simulink model "Avoid_vat_can_3xe"  (R2021b)
settings: Solver=FixedStepAuto  StartTime=0.0  StopTime=40  FixedStep=0.01  RelTol=1e-3
values from neighbouring files (symbols this model uses):
  G_target = [5.8;8.0]    [parameter.m]
  Position_first_vehicle = [Set_first(1);Set_first(2);deg2rad(19.5)]    [parameter.m]
  Q_can = [4.4;7.2]    [parameter.m]
  Set_first = [3;6]    [parameter.m]
settings Model: Creator=HL_1810  LastModifiedBy=HL_1810

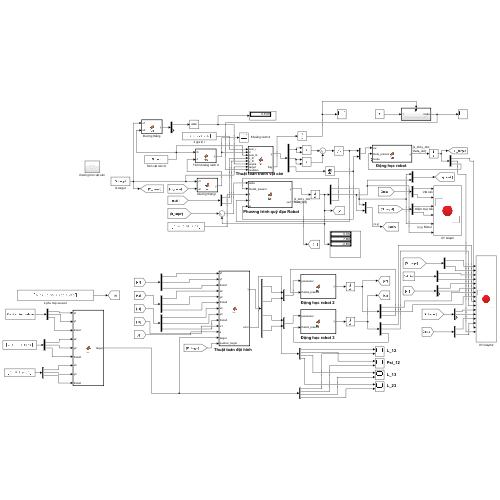
[thumbnail: Simulink's stored preview of the top-level diagram]
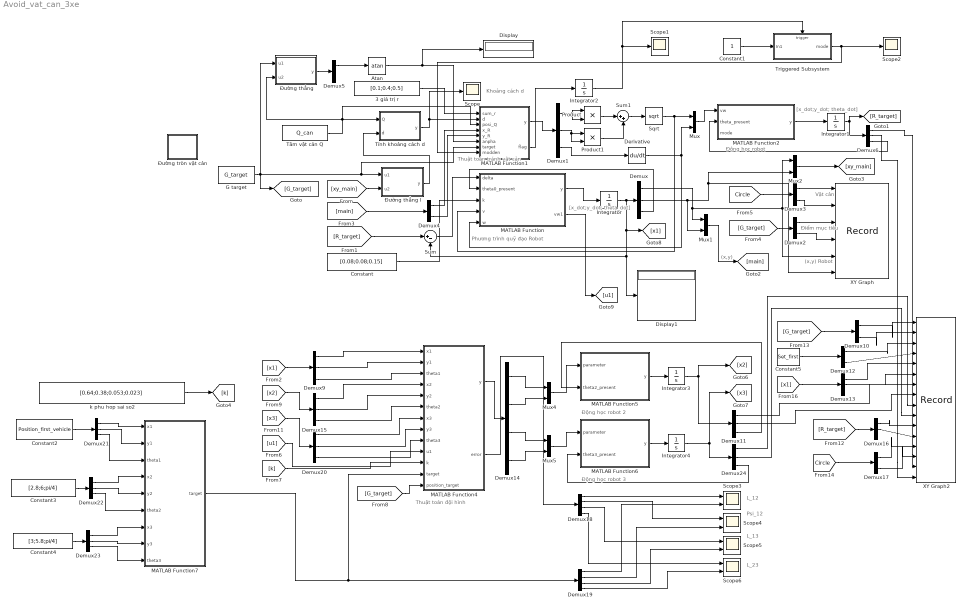
== system Avoid_vat_can_3xe ==
  note: (x,y)
  note: Điểm mục tiêu
  note: (x,y) Robot
  note: Động học robot
  note: Khoảng cách d
  note: Phương trình quỹ đạo Robot
  note: Thuật toán tránh vật cản
  note: Vật cản
  note: [x_dot;y_dot;
      | theta_dot]
  note: [x_dot;y_dot;
      | theta_dot]
  note: L_12
  note: Psi_12
  note: Động học robot 3
  note: L_13
  note: Động học robot 2
  note: L_23
  note: Thuật toán đội hình
  3 giá trị r : Constant  Value=[0.1;0.4;0.5]
  Atan : Trigonometry  Operator=atan
  Constant : Constant  Value=[0.08;0.08;0.15]
  Constant1 : Constant
  Constant2 : Constant  Value=Position_first_vehicle
  Constant3 : Constant  Value=[2.8;6;pi/4]
  Constant4 : Constant  Value=[3;5.8;pi/4]
  Constant5 : Constant  Value=Set_first
  Demux{,1,6,9,11,13,15..16,20..24} (13 alike) : Demux  Outputs=3
  Demux{2..5,10,12,17} (7 alike) : Demux  Outputs=2
  Demux14 : Demux
  Demux18 : Demux
  Demux19 : Demux
  Derivative : Derivative
  Display : Display
  Display1 : Display
  G target : Constant  Value=G_target
  Integrator : Integrator  InitialCondition=Position_first_vehicle
  Integrator1 : Integrator  InitialCondition=Position_first_vehicle
  Integrator2 : Integrator
  Integrator3 : Integrator  InitialCondition=[2.8;6;pi/4]
  Integrator4 : Integrator  InitialCondition=[3;5.8;pi/4]
  MATLAB Function : MATLAB Function  TreatAsAtomicUnit=on
  MATLAB Function1 : MATLAB Function  TreatAsAtomicUnit=on
  MATLAB Function2 : MATLAB Function  TreatAsAtomicUnit=on
  MATLAB Function4 : MATLAB Function  TreatAsAtomicUnit=on
  MATLAB Function5 : MATLAB Function  TreatAsAtomicUnit=on
  MATLAB Function6 : MATLAB Function  TreatAsAtomicUnit=on
  MATLAB Function7 : MATLAB Function  TreatAsAtomicUnit=on
  Mux{,1..2,4..5} (5 alike) : Mux  Inputs=2
  Product : Product
  Product1 : Product
  Scope : Scope
  Scope1 : Scope
  Scope2 : Scope
  Scope{3..6} (4 alike) : Scope  NumInputPorts=2
  Sqrt : Sqrt  SaturateOnIntegerOverflow=on
  Sum : Sum  Inputs=|+-
  Sum1 : Sum  Inputs=|++
  Triggered Subsystem : Subsystem  TreatAsAtomicUnit=on
  Tâm vật cản Q : Constant  Value=Q_can
  Tính khoảng cách d : MATLAB Function  TreatAsAtomicUnit=on
  XY Graph : Record  FileSettingsInternal="{\"entries\":[{\"content\":{\"excelSettings\":{\"content\":{},\"type\":\"Streamout.ExcelSettings\"}},\"type\":\"Streamout.FileSettingStorage\",\"uuid\":\"a8d3b570-9e37-41a1-b9b1-4b418e9d51ca\"}],\"packageUris\":[\"http://schema.mathworks.com/mf0/streamout_blocks/R2020a\"],\"version\":\"1.0\"}"  Layout=[1 1]  SignalsInternal="{\"entries\":[{\"content\":{\"signals\":[{\"content\":{\"blockPath\":[\"Avoid_vat_can_3xe/XY Graph\"],\"channel\":[],\"dimensions\":[1],\"domain\":\"Avoid_vat_can_3xe/XY Graph\",\"lineColor\":\"#ff6929\",\"plots\":[1],\"port\":1,\"sid\":[\"\"],\"signalID\":4338,\"signalName\":\"Demux3:1\"},\"type\":\"RecordBlkView.Signal\",\"uuid\":\"8399b9d0-b1dd-4b64-90be-267014180888\"},{\"content\":{\"blockPath\":[\"Avoid_vat_can_3xe/XY Graph\"],\"channel\":[],\"dimensions\":[1],\"domain\":\"Avoid_vat_can_3xe/XY Graph\",\"lineColor\":\"#b746ff\",\"plots\":[1],\"port\":2,\"sid\":[\"\"],\"signalID\":4342,\"signalName\":\"Demux3:2\"},\"type\":\"RecordBlkView.Signal\",\"uuid\":\"5d023b2a-6e03-4b3e-9db3-6ad99874a4d7\"},{\"content\":{\"blockPath\":[\"Avoid_vat_can_3xe/XY Graph\"],\"channel\":[],\"dimensions\":[1],\"domain\":\"Avoid_vat_can_3xe/XY Graph\",\"lineColor\":\"#64d413\",\"plots\":[1],\"port\":5,\"sid\":[\"\"],\"signalID\":4346,\"signalName\":\"Demux:1\"},\"type\":\"RecordBlkView.Signal\",\"uuid\":\"95680c87-e324-4348-a78d-b81f180a8f94\"},{\"content\":{\"blockPath\":[\"Avoid_vat_can_3xe/XY Graph\"],\"channel\":[],\"dimensions\":[1],\"domain\":\"Avoid_vat_can_3xe/XY Graph\",\"lineColor\":\"#ff13a6\",\"plots\":[1],\"port\":6,\"sid\":[\"\"],\"signalID\":4350,\"signalName\":\"Demux:2\"},\"type\":\"RecordBlkView.Signal\",\"uuid\":\"adc273e3-6312-475d-85d5-afca6bf7d5e4\"},{\"content\":{\"blockPath\":[\"Avoid_vat_can_3xe/XY Graph\"],\"channel\":[],\"dimensions\":[1],\"domain\":\"Avoid_vat_can_3xe/XY Graph\",\"lineColor\":\"#fe330a\",\"plots\":[1],\"port\":3,\"sid\":[\"\"],\"signalID\":4402,\"signalName\":\"Demux2:1\"},\"type\":\"RecordBlkView.Signal\",\"uuid\":\"c6965b63-4477-498a-81ce-133a2781b2ed\"},{\"content\":{\"blockPath\":[\"Avoid_vat_can_3xe/XY Graph\"],\"channel\":[],\"dimensions\":[1],\"domain\":\"Avoid_vat_can_3xe/XY Graph\",\"lineColor\":\"#22b573\",\"plots\":[1],\"port\":4,\"sid\":[\"\"],\"signalID\":4406,\"signalName\":\"Demux2:2\"},\"type\":\"RecordBlkView.Signal\",\"uuid\":\"82515902-e219-45b4-8869-39249660641d\"}]},\"type\":\"RecordBlkView.InputSignals\",\"uuid\":\"3ec44429-ff9f-4d5f-a42a-4439dbfec8c0\"}],\"packageUris\":[\"http://schema.mathworks.com/mf0/streamout_blocks/R2020a\"],\"version\":\"1.0\"}"  VisualizationBindings="{\"xyplotplugin\":{\"info\":[{\"series\":[{\"bindingParametersList\":[{\"parameter\":\"X-Axis\",\"signalID\":4338,\"signalName\":\"Demux3:1\"},{\"parameter\":\"Y-Axis\",\"signalID\":4342,\"signalName\":\"Demux3:2\"}],\"seriesID\":26607},{\"bindingParametersList\":[{\"parameter\":\"X-Axis\",\"signalID\":4402,\"signalName\":\"Demux2:1\"},{\"parameter\":\"Y-Axis\",\"signalID\":4406,\"signalName\":\"Demux2:2\"}],\"seriesID\":58074},{\"bindingParametersList\":[{\"parameter\":\"X-Axis\",\"signalID\":4346,\"signalName\":\"Demux:1\"},{\"parameter\":\"Y-Axis\",\"signalID\":4350,\"signalName\":\"Demux:2\"}],\"seriesID\":51744}],\"subplotID\":1},{\"series\":[],\"subplotID\":2}]}}"  CompatibilityTag=XY
  XY Graph2 : Record  FileSettingsInternal="{\"entries\":[{\"content\":{\"excelSettings\":{\"content\":{},\"type\":\"Streamout.ExcelSettings\"}},\"type\":\"Streamout.FileSettingStorage\",\"uuid\":\"ed37455e-9adf-4e9b-bed2-b0034767e237\"}],\"packageUris\":[\"http://schema.mathworks.com/mf0/streamout_blocks/R2020a\"],\"version\":\"1.0\"}"  Layout=[1 1]  SignalsInternal="{\"entries\":[{\"content\":{\"signals\":[{\"content\":{\"blockPath\":[\"Avoid_vat_can_3xe/XY Graph2\"],\"channel\":[],\"dimensions\":[1],\"domain\":\"Avoid_vat_can_3xe/XY Graph2\",\"lineColor\":\"#ff6929\",\"plots\":[1],\"port\":5,\"sid\":[\"\"],\"signalID\":4354,\"signalName\":\"Demux13:1\"},\"type\":\"RecordBlkView.Signal\",\"uuid\":\"0d8b8474-356b-455b-a3d2-928f594b97db\"},{\"content\":{\"blockPath\":[\"Avoid_vat_can_3xe/XY Graph2\"],\"channel\":[],\"dimensions\":[1],\"domain\":\"Avoid_vat_can_3xe/XY Graph2\",\"lineColor\":\"#b746ff\",\"plots\":[1],\"port\":6,\"sid\":[\"\"],\"signalID\":4358,\"signalName\":\"Demux13:2\"},\"type\":\"RecordBlkView.Signal\",\"uuid\":\"c7b2e1ea-afc6-4af0-a64e-b0961d81559b\"},{\"content\":{\"blockPath\":[\"Avoid_vat_can_3xe/XY Graph2\"],\"channel\":[],\"dimensions\":[1,1],\"domain\":\"Avoid_vat_can_3xe/XY Graph2\",\"lineColor\":\"#64d413\",\"plots\":[1],\"port\":7,\"sid\":[\"\"],\"signalID\":4362,\"signalName\":\"Demux11:1\"},\"type\":\"RecordBlkView.Signal\",\"uuid\":\"9d6d36d3-8fd9-4190-aa51-39a149636880\"},{\"content\":{\"blockPath\":[\"Avoid_vat_can_3xe/XY Graph2\"],\"channel\":[],\"dimensions\":[1,1],\"domain\":\"Avoid_vat_can_3xe/XY Graph2\",\"lineColor\":\"#ff13a6\",\"plots\":[1],\"port\":8,\"sid\":[\"\"],\"signalID\":4366,\"signalName\":\"Demux11:2\"},\"type\":\"RecordBlkView.Signal\",\"uuid\":\"809edec6-6648-46b3-b799-dc7e2610b91b\"},{\"content\":{\"blockPath\":[\"Avoid_vat_can_3xe/XY Graph2\"],\"channel\":[],\"dimensions\":[1,1],\"domain\":\"Avoid_vat_can_3xe/XY Graph2\",\"lineColor\":\"#fe330a\",\"plots\":[1],\"port\":9,\"sid\":[\"\"],\"signalID\":4370,\"signalName\":\"Demux24:1\"},\"type\":\"RecordBlkView.Signal\",\"uuid\":\"bc8e87cb-6b4d-42b2-8550-ea17e29acf2f\"},{\"content\":{\"blockPath\":[\"Avoid_vat_can_3xe/XY Graph2\"],\"channel\":[],\"dimensions\":[1,1],\"domain\":\"Avoid_vat_can_3xe/XY Graph2\",\"lineColor\":\"#22b573\",\"plots\":[1],\"port\":10,\"sid\":[\"\"],\"signalID\":4374,\"signalName\":\"Demux24:2\"},\"type\":\"RecordBlkView.Signal\",\"uuid\":\"436826c5-510a-4675-9b17-c630ed9073da\"},{\"content\":{\"blockPath\":[\"Avoid_vat_can_3xe/XY Graph2\"],\"channel\":[],\"dimensions\":[1],\"domain\":\"Avoid_vat_can_3xe/XY Graph2\",\"lineColor\":\"#0072bd\",\"plots\":[1],\"port\":11,\"sid\":[\"\"],\"signalID\":4378,\"signalName\":\"Demux16:1\"},\"type\":\"RecordBlkView.Signal\",\"uuid\":\"45a9fc4d-343a-4103-b6bd-5c0be15f774b\"},{\"content\":{\"blockPath\":[\"Avoid_vat_can_3xe/XY Graph2\"],\"channel\":[],\"dimensions\":[1],\"domain\":\"Avoid_vat_can_3xe/XY Graph2\",\"lineColor\":\"#d95319\",\"plots\":[1],\"port\":12,\"sid\":[\"\"],\"signalID\":4382,\"signalName\":\"Demux16:2\"},\"type\":\"RecordBlkView.Signal\",\"uuid\":\"679dac8d-d637-4fab-bff7-509533d3bec0\"},{\"content\":{\"blockPath\":[\"Avoid_vat_can_3xe/XY Graph2\"],\"channel\":[],\"dimensions\":[1],\"domain\":\"Avoid_vat_can_3xe/XY Graph2\",\"lineColor\":\"#fe330a\",\"plots\":[1],\"port\":13,\"sid\":[\"\"],\"signalID\":4386,\"signalName\":\"Demux17:1\"},\"type\":\"RecordBlkView.Signal\",\"uuid\":\"4ab9b0f9-b6f9-4618-a1ff-eb8b4a502663\"},{\"content\":{\"blockPath\":[\"Avoid_vat_can_3xe/XY Graph2\"],\"channel\":[],\"dimensions\":[1],\"domain\":\"Avoid_vat_can_3xe/XY Graph2\",\"lineColor\":\"#22b573\",\"plots\":[1],\"port\":14,\"sid\":[\"\"],\"signalID\":4390,\"signalName\":\"Demux17:2\"},\"type\":\"RecordBlkView.Signal\",\"uuid\":\"5823eff9-447f-4ca4-82e1-f72dafea7aa2\"},{\"content\":{\"blockPath\":[\"Avoid_vat_can_3xe/XY Graph2\"],\"channel\":[],\"dimensions\":[1],\"domain\":\"Avoid_vat_can_3xe/XY Graph2\",\"lineColor\":\"#64d413\",\"plots\":[1],\"port\":15,\"sid\":[\"\"],\"signalID\":4394,\"signalName\":\"Demux6:1\"},\"type\":\"RecordBlkView.Signal\",\"uuid\":\"6e0b1d86-1497-48ad-b697-da4d1b4b05da\"},{\"content\":{\"blockPath\":[\"Avoid_vat_can_3xe/XY Graph2\"],\"channel\":[],\"dimensions\":[1],\"domain\":\"Avoid_vat_can_3xe/XY Graph2\",\"lineColor\":\"#ff13a6\",\"plots\":[1],\"port\":16,\"sid\":[\"\"],\"signalID\":4398,\"signalName\":\"Demux6:2\"},\"type\":\"RecordBlkView.Signal\",\"uuid\":\"a773829a-94af-4e1e-bb77-84491575b248\"},{\"content\":{\"blockPath\":[\"Avoid_vat_can_3xe/XY Graph2\"],\"channel\":[],\"dimensions\":[1],\"domain\":\"Avoid_vat_can_3xe/XY Graph2\",\"lineColor\":\"#77ac30\",\"plots\":[1],\"port\":1,\"sid\":[\"\"],\"signalID\":4410,\"signalName\":\"Demux10:1\"},\"type\":\"RecordBlkView.Signal\",\"uuid\":\"59508f2c-7fd3-4530-ba17-a0911d246959\"},{\"content\":{\"blockPath\":[\"Avoid_vat_can_3xe/XY Graph2\"],\"channel\":[],\"dimensions\":[1],\"domain\":\"Avoid_vat_can_3xe/XY Graph2\",\"lineColor\":\"#4dbeee\",\"plots\":[1],\"port\":2,\"sid\":[\"\"],\"signalID\":4414,\"signalName\":\"Demux10:2\"},\"type\":\"RecordBlkView.Signal\",\"uuid\":\"ec991bf2-35d2-4910-97d5-0e3210c8fdc5\"},{\"content\":{\"blockPath\":[\"Avoid_vat_can_3xe/XY Graph2\"],\"channel\":[],\"dimensions\":[1],\"domain\":\"Avoid_vat_can_3xe/XY Graph2\",\"lineColor\":\"#a2142f\",\"plots\":[1],\"port\":3,\"sid\":[\"\"],\"signalID\":4418,\"signalName\":\"Demux12:1\"},\"type\":\"RecordBlkView.Signal\",\"uuid\":\"ee91cbce-6ec2-4539-97e0-c14b3cec1737\"},{\"content\":{\"blockPath\":[\"Avoid_vat_can_3xe/XY Graph2\"],\"channel\":[],\"dimensions\":[1],\"domain\":\"Avoid_vat_can_3xe/XY Graph2\",\"lineColor\":\"#139fff\",\"plots\":[1],\"port\":4,\"sid\":[\"\"],\"signalID\":4422,\"signalName\":\"Demux12:2\"},\"type\":\"RecordBlkView.Signal\",\"uuid\":\"70b86e27-9af5-45e0-b5a5-07d061f29a2f\"}]},\"type\":\"RecordBlkView.InputSignals\",\"uuid\":\"da098691-6c74-41c8-987e-b431dd933fcf\"}],\"packageUris\":[\"http://schema.mathworks.com/mf0/streamout_blocks/R2020a\"],\"version\":\"1.0\"}"  VisualizationBindings="{\"xyplotplugin\":{\"info\":[{\"series\":[{\"bindingParametersList\":[{\"parameter\":\"X-Axis\",\"signalID\":4410,\"signalName\":\"Demux10:1\"},{\"parameter\":\"Y-Axis\",\"signalID\":4414,\"signalName\":\"Demux10:2\"}],\"seriesID\":62746},{\"bindingParametersList\":[{\"parameter\":\"X-Axis\",\"signalID\":4386,\"signalName\":\"Demux17:1\"},{\"parameter\":\"Y-Axis\",\"signalID\":4390,\"signalName\":\"Demux17:2\"}],\"seriesID\":60584},{\"bindingParametersList\":[{\"parameter\":\"X-Axis\",\"signalID\":4362,\"signalName\":\"Demux11:1\"},{\"parameter\":\"Y-Axis\",\"signalID\":4366,\"signalName\":\"Demux11:2\"}],\"seriesID\":48459},{\"bindingParametersList\":[{\"parameter\":\"X-Axis\",\"signalID\":4354,\"signalName\":\"Demux13:1\"},{\"parameter\":\"Y-Axis\",\"signalID\":4358,\"signalName\":\"Demux13:2\"}],\"seriesID\":55138},{\"bindingParametersList\":[{\"parameter\":\"X-Axis\",\"signalID\":4370,\"signalName\":\"Demux24:1\"},{\"parameter\":\"Y-Axis\",\"signalID\":4374,\"signalName\":\"Demux24:2\"}],\"seriesID\":43364},{\"bindingParametersList\":[{\"parameter\":\"X-Axis\",\"signalID\":4378,\"signalName\":\"Demux16:1\"},{\"parameter\":\"Y-Axis\",\"signalID\":4382,\"signalName\":\"Demux16:2\"}],\"seriesID\":33810},{\"bindingParametersList\":[{\"parameter\":\"X-Axis\",\"signalID\":4418,\"signalName\":\"Demux12:1\"},{\"parameter\":\"Y-Axis\",\"signalID\":4422,\"signalName\":\"Demux12:2\"}],\"seriesID\":55166},{\"bindingParametersList\":[{\"parameter\":\"X-Axis\",\"signalID\":4394,\"signalName\":\"Demux6:1\"},{\"parameter\":\"Y-Axis\",\"signalID\":4398,\"signalName\":\"Demux6:2\"}],\"seriesID\":47059}],\"subplotID\":1},{\"series\":[],\"subplotID\":2},{\"series\":[],\"subplotID\":9},{\"series\":[],\"subplotID\":10}]}}"  CompatibilityTag=XY
  k phu hop sai so2 : Constant  Value=[0.64;0.38;0.053;0.023]
  Đường thẳng : MATLAB Function  TreatAsAtomicUnit=on
  "Đường thẳng l " : MATLAB Function  TreatAsAtomicUnit=on
  Đường tròn vật cản : Subsystem
  wires:
  MATLAB Function2/1(y) -> Integrator1/1
  Integrator2/1 -> Triggered Subsystem/Trigger, Scope1/1
  [R_target] -> Sum/1
  Mux/1 -> MATLAB Function2/1(vw)
  Demux3/2 -> XY Graph/2
  Demux1/3 -> Derivative/1
  Demux4/1 -> MATLAB Function1/4(x_R)
  Demux3/1 -> XY Graph/1
  Tính khoảng cách d/1(y) -> Scope/1, MATLAB Function1/2(d)
  [G_target] -> Demux2/1
  MATLAB Function/1(y) -> Integrator/1
  Tâm vật cản Q/1 -> Tính khoảng cách d/1(Q), Đường thẳng/2(u2), MATLAB Function1/3(posi_Q)
  3 giá trị r/1 -> MATLAB Function1/1(sum_r)
  Sqrt/1 -> Mux/1, MATLAB Function/4(v)
  MATLAB Function1/2(flag) -> Integrator2/1
  Demux1/1 -> Product/2, Product/1
  [xy_main] -> "Đường thẳng l "/2(u2)
  Constant/1 -> MATLAB Function/3(k)
  Demux5/1 -> Atan/1
  Atan/1 -> Display/1, MATLAB Function1/6(anpha)
  [main] -> Demux4/1
  Mux1/1 -> [main]
  Derivative/1 -> MATLAB Function/5(w), Mux/2
  Triggered Subsystem/1(mode) -> MATLAB Function1/8(modden), Scope2/1
  Demux/3 -> MATLAB Function/2(theta0_present)
  Integrator1/1 -> Demux6/1, [R_target]
  Demux4/2 -> MATLAB Function1/5(y_R)
  Demux2/1 -> XY Graph/3
  [Circle] -> Demux3/1
  "Đường thẳng l "/1(y) -> Tính khoảng cách d/2(d)
  Demux6/3 -> MATLAB Function2/2(theta_present)
  Sum1/1 -> Sqrt/1
  Product/1 -> Sum1/1
  Integrator/1 -> Demux/1, [x1], Display1/1, Sum/2
  Mux2/1 -> [xy_main]
  Demux/1 -> XY Graph/5, Mux2/1, Mux1/1
  Demux/2 -> Mux1/2, XY Graph/6, Mux2/2
  Demux1/2 -> Product1/2, Product1/1
  Demux2/2 -> XY Graph/4
  Constant1/1 -> Triggered Subsystem/1(In1)
  Product1/1 -> Sum1/2
  Đường thẳng/1(y) -> Demux5/1
  G target/1 -> [G_target], Đường thẳng/1(u1), MATLAB Function1/7(target), "Đường thẳng l "/1(u1)
  Sum/1 -> MATLAB Function/1(delta)
  MATLAB Function1/1(y) -> Demux1/1
  Demux14/4 -> Mux5/2
  Demux9/2 -> MATLAB Function4/2(y1)
  Integrator4/1 -> Demux24/1, [x3]
  Demux20/3 -> MATLAB Function4/9(theta3)
  Demux19/1 -> Scope3/2
  Demux23/2 -> MATLAB Function7/8(y3)
  Demux23/1 -> MATLAB Function7/7(x3)
  Constant4/1 -> Demux23/1
  Constant3/1 -> Demux22/1
  MATLAB Function7/1(target) -> MATLAB Function4/12(target), Demux19/1
  Demux19/4 -> Scope6/2
  Demux11/3 -> MATLAB Function5/2(theta2_present)
  [G_target] -> Demux10/1
  Demux20/2 -> MATLAB Function4/8(y3)
  Demux21/1 -> MATLAB Function7/1(x1)
  Demux15/2 -> MATLAB Function4/5(y2)
  Demux23/3 -> MATLAB Function7/9(theta3)
  Demux22/2 -> MATLAB Function7/5(y2)
  [R_target] -> Demux16/1
  Demux22/1 -> MATLAB Function7/4(x2)
  Demux21/2 -> MATLAB Function7/2(y1)
  Demux22/3 -> MATLAB Function7/6(theta2)
  Constant2/1 -> Demux21/1
  [x2] -> Demux15/1
  Demux11/2 -> XY Graph2/8
  Demux10/2 -> XY Graph2/2
  Demux10/1 -> XY Graph2/1
  Demux12/1 -> XY Graph2/3
  [x1] -> Demux9/1
  Demux24/3 -> MATLAB Function6/2(theta3_present)
  Demux9/1 -> MATLAB Function4/1(x1)
  Demux14/2 -> Mux4/2
  Mux5/1 -> MATLAB Function6/1(parameter)
  Demux20/1 -> MATLAB Function4/7(x3)
  MATLAB Function4/1(y) -> Demux14/1
  Demux24/1 -> XY Graph2/9
  Integrator3/1 -> Demux11/1, [x2]
  MATLAB Function4/2(error) -> Demux18/1
  Demux13/2 -> XY Graph2/6
  [x1] -> Demux13/1
  Demux14/3 -> Mux5/1
  Demux9/3 -> MATLAB Function4/3(theta1)
  Demux12/2 -> XY Graph2/4
  Demux14/1 -> Mux4/1
  [x3] -> Demux20/1
  Demux15/1 -> MATLAB Function4/4(x2)
  Demux18/4 -> Scope6/1
  MATLAB Function5/1(y) -> Integrator3/1
  [Circle] -> Demux17/1
  Demux18/3 -> Scope5/1
  Demux17/1 -> XY Graph2/13
  Demux11/1 -> XY Graph2/7
  Demux18/1 -> Scope3/1
  Constant5/1 -> Demux12/1
  Demux19/3 -> Scope5/2
  Demux21/3 -> MATLAB Function7/3(theta1)
  Demux19/2 -> Scope4/2
  Demux18/2 -> Scope4/1
  Demux24/2 -> XY Graph2/10
  Demux17/2 -> XY Graph2/14
  Demux15/3 -> MATLAB Function4/6(theta2)
  Demux13/1 -> XY Graph2/5
  Demux16/1 -> XY Graph2/11
  [k] -> MATLAB Function4/11(k)
  Mux4/1 -> MATLAB Function5/1(parameter)
  [u1] -> MATLAB Function4/10(u1)
  MATLAB Function6/1(y) -> Integrator4/1
  Demux16/2 -> XY Graph2/12
  MATLAB Function/2(vw1) -> [u1]
  k phu hop sai so2/1 -> [k]
  [G_target] -> MATLAB Function4/13(position_target)
  Demux6/1 -> XY Graph2/15
  Demux6/2 -> XY Graph2/16

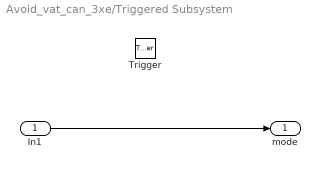
== system Avoid_vat_can_3xe/Triggered Subsystem ==
  In1 : Inport
  Trigger : TriggerPort  VariantControl=(inherit)
  mode : Outport
  wires:
  In1/1 -> mode/1

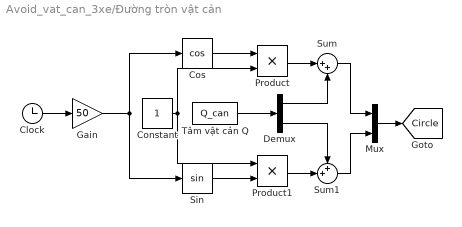
== system Avoid_vat_can_3xe/Đường tròn vật cản ==
  Clock : Clock
  Constant : Constant
  Cos : Trigonometry  Operator=cos
  Demux : Demux  Outputs=2
  Gain : Gain  Gain=50
  Mux : Mux  Inputs=2
  Product : Product
  Product1 : Product
  Sin : Trigonometry
  Sum : Sum  Inputs=|++
  Sum1 : Sum  Inputs=++|
  Tâm vật cản Q : Constant  Value=Q_can
  tag scope: Circle=global
  wires:
  Product1/1 -> Sum1/2
  Constant/1 -> Product1/1, Product/2
  Product/1 -> Sum/1
  Sum/1 -> Mux/1
  Cos/1 -> Product/1
  Sum1/1 -> Mux/2
  Mux/1 -> [Circle]
  Clock/1 -> Gain/1
  Gain/1 -> Sin/1, Cos/1
  Sin/1 -> Product1/2
  Tâm vật cản Q/1 -> Demux/1
  Demux/1 -> Sum/2
  Demux/2 -> Sum1/1

== matlab function Avoid_vat_can_3xe/MATLAB Function5 ==
  data: parameter input; y output; theta2_present input
function y = fcn(parameter,theta2_present)
%#codegen
Matrix=[cos(theta2_present) 0;
        sin(theta2_present) 0;
        0                   1];
u=Matrix*parameter;
y = u;

== matlab function Avoid_vat_can_3xe/MATLAB Function6 ==
  data: parameter input; y output; theta3_present input
function y = fcn(parameter,theta3_present)
%#codegen
Matrix=[cos(theta3_present) 0;
        sin(theta3_present) 0;
        0                   1];
u=Matrix*parameter;
y = u;

== matlab function Avoid_vat_can_3xe/MATLAB Function7 ==
  data: x1 input; target output; y1 input; theta1 input; x2 input; y2 input; theta2 input; x3 input; y3 input; theta3 input
function target = fcn(x1,y1,theta1,x2,y2,theta2,x3,y3,theta3)
%#codegen
d=0.09;

L12_x=x1-x2-d*cos(theta2);
L12_y=y1-y2-d*sin(theta2);
L13_x=x1-x3-d*cos(theta3);
L13_y=y1-y3-d*sin(theta3);
L23_x=x2-x3-d*cos(theta3);
L23_y=y2-y3-d*sin(theta3);

L12=sqrt(L12_x^2+L12_y^2);
L13=sqrt(L13_x^2+L13_y^2);
L23=sqrt(L23_x^2+L23_y^2);

mega12=atan(L12_y/L12_x)-theta1+pi;
target=[L12;mega12;L13;L23];

== matlab function Avoid_vat_can_3xe/Đường thẳng l  ==
  data: u1 input; y output; u2 input
function y = fcn(u1,u2)
%#codegen
% Đường thẳng từ tâm Robot đến điểm mục tiêu
a=(u1(2)-u2(2))/(u1(1)-u2(1));
b=u1(2)-u1(1)*a;
u=[a;b];
y = u;

== matlab function Avoid_vat_can_3xe/MATLAB Function ==
  data: delta input; y output; theta0_present input; k input; v input; w input; vw1 output
function [y,vw1] = fcn(delta,theta0_present,k,v,w)
%#codegen
A=[cos(theta0_present)   sin(theta0_present) 0;
    -sin(theta0_present) cos(theta0_present) 0;
    0                    0                    1];
e=A*delta;
V_c=[v*cos(e(3))+k(1)*e(1);
    w+k(2)*v*e(2)+k(3)*v*sin(e(3))];

Matrix=[cos(theta0_present) 0;
        sin(theta0_present) 0;
        0                   1];
u=Matrix*V_c;
vw1=V_c;
y = u;

== matlab function Avoid_vat_can_3xe/Tính khoảng cách d ==
  data: Q input; y output; d input
function y = fcn(Q,d)
%#codegen
a=d(1);
b=-1;
c=d(2);
u=( Q(1)*a + b*Q(2) +c )/sqrt(a^2+b^2);
y = u;

== matlab function Avoid_vat_can_3xe/MATLAB Function1 ==
  data: sum_r input; y output; d input; posi_Q input; x_R input; y_R input; anpha input; target input; flag output; modden input
function [y,flag]= fcn(sum_r,d,posi_Q,x_R,y_R,anpha,target,modden)
%#codegen
rv=sum_r(1)+sum_r(2)+sum_r(3);



M=[cos(anpha) -sin(anpha) 0 posi_Q(1);
    sin(anpha) cos(anpha) 0 posi_Q(2);
    0 0 1 0;
    0 0 0 1];
N=[x_R;y_R;0;1];
Vitri=inv(M)*N;
dd=abs(2.4843*x_R-y_R-6.4)/sqrt(2.4843^2+1);
if ((d<rv) &&(dd>0.01))
    mode=0;
else
    mode=1;

end

if (modden==0)
        xr_dot=(d/abs(d))*Vitri(2)+Vitri(1)*(rv^2-Vitri(1)^2-Vitri(2)^2);
        yr_dot=-(d/abs(d))*Vitri(1)+Vitri(2)*(rv^2-Vitri(1)^2-Vitri(2)^2);
        theta_r=atan(yr_dot/xr_dot);
else
    if ((x_R-target(1))^2+(y_R-target(2))^2) > 0.001
            xr_dot = 0.04*cos(atan((y_R)-target(2))/((x_R)-target(1)));
            yr_dot = 0.04*sin(atan((y_R)-target(2))/((x_R)-target(1)));
            theta_r = atan((y_R)-target(2))/((x_R)-target(1));
        else 
            xr_dot = 0;
            yr_dot = 0;
            theta_r =0 ;
    end
end



u=[xr_dot;yr_dot;theta_r];

y = u;
flag=mode;

== matlab function Avoid_vat_can_3xe/MATLAB Function2 ==
  data: vw input; y output; theta_present input; mode input
function y = fcn(vw,theta_present,mode)
%#codegen
% if (mode==0)
%     vw1=[vw(1);vw(2)];
% else
%     vw1=[0.04;0];
% end
Matrix=[cos(theta_present) 0;
        sin(theta_present) 0;
        0                   1];
u=Matrix*vw;
y = u;

== matlab function Avoid_vat_can_3xe/Đường thẳng ==
  data: u1 input; y output; u2 input
function y = fcn(u1,u2)
%Đường thẳng từ mục tiêu đến tâm vật cản
a=(u1(2)-u2(2))/(u1(1)-u2(1)); %hệ số góc
b=u1(2)-u1(1)*a;
u=[a;b];
y = u;

== matlab function Avoid_vat_can_3xe/MATLAB Function4 ==
  data: x1 input; y output; y1 input; theta1 input; x2 input; y2 input; theta2 input; x3 input; y3 input; theta3 input; u1 input; k input; target input; error output; position_target input
function [y,error] = fcn(x1,y1,theta1,x2,y2,theta2,x3,y3,theta3,u1,k,target,position_target)
%#codegen
d=0.09;

L12_x=x1-x2-d*cos(theta2);
L12_y=y1-y2-d*sin(theta2);
L13_x=x1-x3-d*cos(theta3);
L13_y=y1-y3-d*sin(theta3);
L23_x=x2-x3-d*cos(theta3);
L23_y=y2-y3-d*sin(theta3);

L12=sqrt(L12_x^2+L12_y^2);
L13=sqrt(L13_x^2+L13_y^2);
L23=sqrt(L23_x^2+L23_y^2);

mega12=atan(L12_y/L12_x)-theta1+pi;
mega13=atan(L13_y/L13_x)-theta1+pi;
mega23=atan(L23_y/L23_x)-theta2+pi;

beta12=theta1-theta2;
beta13=theta1-theta3;
beta23=theta2-theta3;

si12=beta12+mega12;
si13=beta13+mega13;
si23=beta23+mega23;

G2=[cos(si12)      d*sin(si12)     0         0;
    -sin(si12)/L12 d*cos(si12)/L12 0         0;
    0              0               cos(si13) d*sin(si13);
    -cos(mega23)   0               cos(si23) d*sin(si23)];

F2=[-cos(mega12)     0;
    sin(mega12)/L12 -1;
    -cos(mega13)     0;
    0                0];
p= [k(1)*(target(1)-L12);
    k(2)*(target(2)-mega12);
    k(3)*(target(3)-L13);
    k(4)*(target(4)-L23)];
e=[L12;
mega12;
L13;
L23];
if (sqrt((position_target(1)-x1)^2+(position_target(2)-y1)^2)>=0.05)
    u=inv(G2)*(p-F2*u1);
else
    u=[0;0;0;0];
end
error=e;
y = u;
